simulink model "subsystem_118_bus"  (R2025b)
settings: Solver=ode45  StartTime=0.0  StopTime=Tstop  FixedStep=Ts  RelTol=1e-12  AbsTol=1e-12
values from neighbouring files (symbols this model uses):
  Imax = 15    [config_file.m]
  nominalInter =     [nominalInter.mat]
  nominalU =     [nominalU.mat]
  nominalY =     [nominalY.mat]
  sub = struct    [main_sub_118_bus.m]
  sys_j = sys_j(1:end-1)    [IBR_modelGenerator.m]
  sys_j_AA = sys_j    [modularMOR_main.m]
  sys_j_BT = sys_j    [modularMOR_main.m]
  Tstep_gfl = 0.1    [main_sub_118_bus.m]
  Tstep_gfm = 0.1    [main_sub_118_bus.m]
  w = 2*pi*50    (= 314.159265359)    [config_file.m]    (also in mirrorMimoWeightedFrequencyData.m = w(:); modularMOR_main.m = w(:).'; plotTest.m = w(:).')
undefined symbols (not defined in the file or in its folder): con_sub, linSys1, linSys2, linSys3
libraries: simulink x10
(part 3 of 6)

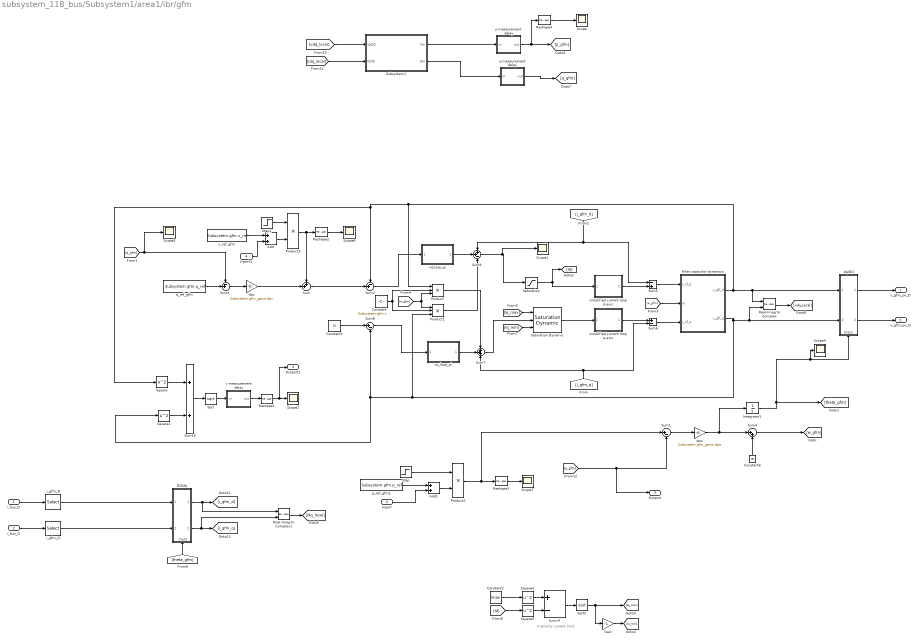
== system subsystem_118_bus/Subsystem1/area1/ibr/gfm ==
  note: P-priority current limit
  i_bus_D : Inport
  i_bus_Q : Inport  Port=2
  Inport : Inport  Port=3
  Inport1 : Inport  Port=4
  Add : Sum
  Add1 : Sum
  Constant : Constant  Value=Subsystem.gfm.c
  Constant1 : Constant  Value=0
  Constant2 : Constant  Value=Imax
  Constant6 : Constant  Value=w
  DQ/dq : Subsystem
      settings: PortSchema="{\"entries\":[{\"content\":{\"sides\":[{\"content\":{\"connectorIds\":[\"In1\",\"In2\"]},\"type\":\"ConnectorPlacement.EquallySpacedRectSide\",\"uuid\":\"6aba5a73-e9d3-440a-9da8-5b4060b79a22\"},{\"content\":{\"connectorIds\":[\"Out1\",\"Out2\"],\"side\":\"RIGHT\"},\"type\":\"ConnectorPlacement.EquallySpacedRectSide\",\"uuid\":\"fb100e33-0f2b-446b-b234-6a01cff1cf94\"},{\"content\":{\"connectorIds\":[],\"side\":\"TOP\"},\"type\":\"ConnectorPlacement.EquallySpacedRectSide\",\"uuid\":\"cb346bab-8363-4920-b8bd-1af08716b150\"},{\"content\":{\"connectorIds\":[\"In3\"],\"side\":\"BOTTOM\"},\"type\":\"ConnectorPlacement.EquallySpacedRectSide\",\"uuid\":\"daf67601-a33f-44c6-bbbf-d32eadf086e5\"},{\"content\":{\"connectorIds\":[],\"side\":\"HIDDEN\"},\"type\":\"ConnectorPlacement.EquallySpacedRectSide\",\"uuid\":\"157b31a2-d1ec-4854-8b21-1495795af5ef\"}]},\"type\":\"ConnectorPlacement.EquallySpacedConnector\",\"uuid\":\"bdcd0df2-60ef-4202-9e13-560935cf5e64\"}],\"packageUris\":[\"http://schema.mathworks.com/mf0/Connector/R2020b\"],\"version\":\"1.0\"}"
      mask Display: image('$imagefile'); % Use "Edit Image" on toolstrip to change.
  Gain : Gain  Gain=-1
  Integrator1 : Integrator  InitialCondition=Subsystem.gfm.theta  ContinuousStateAttributes='gfm_osc'
  Product : Product  Inputs=3
  Product1 : Product  Inputs=3
  Product2 : Product
  Product3 : Product
  Real-Imag to Complex : RealImagToComplex
  Real-Imag to Complex1 : RealImagToComplex
  Reshape{1..4} (4 alike) : Reshape
  Saturation : Saturate  UpperLimit=Imax  LowerLimit=-Imax
  Saturation Dynamic : simulink/Discontinuities/Saturation Dynamic  OutMin=[]  OutMax=[]  OutDataTypeStr=Inherit: Same as second input  OutDataType=fixdt(1, 16)  OutScaling=2^-10  DoSatur=off
  Scope{,1..2,4..5,7..8} (7 alike) : Scope
      Scope settings: ActiveDisplayYMinimum=-1  ActiveDisplayYMaximum=1  DataLoggingVariableName=pm_gfm  DataLoggingSaveFormat=Structure
      Scope1 settings: ActiveDisplayYMinimum=0.57567  ActiveDisplayYMaximum=1.70344
      Scope2 settings: ActiveDisplayYMinimum=1.02215  ActiveDisplayYMaximum=1.04295  DataLoggingVariableName=vm_gfm  DataLoggingSaveFormat=Structure
      Scope4 settings: ActiveDisplayYMinimum=-1  ActiveDisplayYMaximum=1  DataLoggingVariableName=thetagfmwnd  DataLoggingSaveFormat=Structure
      Scope5 settings: ActiveDisplayYMinimum=0.85975274896238685  ActiveDisplayYMaximum=1.0032219511840634  DataLoggingVariableName=qgfmwnd  DataLoggingSaveFormat=Structure
      Scope7 settings: ActiveDisplayYMinimum=-1  ActiveDisplayYMaximum=1  DataLoggingVariableName=pr_gfm  DataLoggingSaveFormat=Structure
      Scope8 settings: ActiveDisplayYMinimum=0.040000000000000036  ActiveDisplayYMaximum=2.04  DataLoggingVariableName=vr_gfm  DataLoggingSaveFormat=Structure
  Sqrt : Sqrt
  Sqrt2 : Sqrt
  Square{,1,4..5} (4 alike) : Math  Operator=square
  Step : Step  Time=Tstep_gfm  Before=Subsystem.P_before_gfm  After=Subsystem.P_after_gfm
  Step1 : Step  Time=Tstep_gfm  Before=Subsystem.V_before_gfm  After=Subsystem.V_after_gfm
  Subsystem1 : Subsystem
      mask Display: image('$imagefile'); % Use "Edit Image" on toolstrip to change.
  Sum : Sum  Inputs=++|
  Sum1 : Sum  Inputs=|+-
  Sum10 : Sum
  Sum14 : Sum  Inputs=+-
  Sum2 : Sum  Inputs=-+|
  Sum3 : Sum  Inputs=-+|
  Sum4 : Sum  Inputs=|++
  Sum5 : Sum  Inputs=-+
  Sum6 : Sum  Inputs=+-
  Sum7 : Sum  Inputs=+++
  Sum8 : Sum  Inputs=|+-
  Sum9 : Sum  Inputs=++-
  dpw : Gain  Gain=Subsystem.gfm_gains.dpw
  dq/DQ : Subsystem
      settings: PortSchema="{\"entries\":[{\"content\":{\"sides\":[{\"content\":{\"connectorIds\":[\"In1\",\"In2\"]},\"type\":\"ConnectorPlacement.EquallySpacedRectSide\",\"uuid\":\"6aba5a73-e9d3-440a-9da8-5b4060b79a22\"},{\"content\":{\"connectorIds\":[\"Out1\",\"Out2\"],\"side\":\"RIGHT\"},\"type\":\"ConnectorPlacement.EquallySpacedRectSide\",\"uuid\":\"fb100e33-0f2b-446b-b234-6a01cff1cf94\"},{\"content\":{\"connectorIds\":[],\"side\":\"TOP\"},\"type\":\"ConnectorPlacement.EquallySpacedRectSide\",\"uuid\":\"cb346bab-8363-4920-b8bd-1af08716b150\"},{\"content\":{\"connectorIds\":[\"In3\"],\"side\":\"BOTTOM\"},\"type\":\"ConnectorPlacement.EquallySpacedRectSide\",\"uuid\":\"daf67601-a33f-44c6-bbbf-d32eadf086e5\"},{\"content\":{\"connectorIds\":[],\"side\":\"HIDDEN\"},\"type\":\"ConnectorPlacement.EquallySpacedRectSide\",\"uuid\":\"157b31a2-d1ec-4854-8b21-1495795af5ef\"}]},\"type\":\"ConnectorPlacement.EquallySpacedConnector\",\"uuid\":\"bdcd0df2-60ef-4202-9e13-560935cf5e64\"}],\"packageUris\":[\"http://schema.mathworks.com/mf0/Connector/R2020b\"],\"version\":\"1.0\"}"
      mask Display: image('$imagefile'); % Use "Edit Image" on toolstrip to change.
  dqv : Gain  Gain=Subsystem.gfm_gains.dqv
  filter capacitor dynamics : Subsystem
      mask Display: image('$imagefile'); % Use "Edit Image" on toolstrip to change.
  i_gfm_D : Selector  InputPortWidth=size(Subsystem.sys_data,1)  IndexOptions=Index vector (dialog)  Indices=Subsystem.busnum.gfm  OutputSizes=1
  i_gfm_Q : Selector  InputPortWidth=size(Subsystem.sys_data,1)  IndexOptions=Index vector (dialog)  Indices=Subsystem.busnum.gfm  OutputSizes=1
  p measurement delay : Subsystem
      mask Display: image('$imagefile'); % Use "Edit Image" on toolstrip to change.
  p_ref_gfm1 : Constant  Value=Subsystem.gfm.p_ref
  q measurement delay : Subsystem
      mask Display: image('$imagefile'); % Use "Edit Image" on toolstrip to change.
  q_ref_gfm : Constant  Value=Subsystem.gfm.q_ref
  simplified current loop d-axis : Subsystem
      mask Display: image('$imagefile'); % Use "Edit Image" on toolstrip to change.
  simplified current loop q-axis : Subsystem
      mask Display: image('$imagefile'); % Use "Edit Image" on toolstrip to change.
  v measurement delay : Subsystem
      mask Display: image('$imagefile'); % Use "Edit Image" on toolstrip to change.
  v_ref_gfm : Constant  Value=Subsystem.gfm.v_ref
  vd_loop_pi : Subsystem
      mask Display: image('$imagefile'); % Use "Edit Image" on toolstrip to change.
  vq_loop_pi : Subsystem
      mask Display: image('$imagefile'); % Use "Edit Image" on toolstrip to change.
  v_gfm_pv_D : Outport
  v_gfm_pv_Q : Outport  Port=2
  Outport : Outport  Port=3
  Outport1 : Outport  Port=4
  wires:
  Sum2/1 -> vd_loop_pi/1("  ")
  dq/DQ/1(D-quantity) -> v_gfm_pv_D/1
  dq/DQ/2(Q-quantity) -> v_gfm_pv_Q/1
  dpw/1 -> Sum4/1, Integrator1/1
  [p_gfm] -> Outport/1, Sum1/2
  Constant6/1 -> Sum4/2
  Sum1/1 -> dpw/1
  Integrator1/1 -> [theta_gfm], Scope4/1, dq/DQ/3(theta)
  Sum/1 -> Sum2/2
  dqv/1 -> Sum/2
  Sum3/1 -> dqv/1
  q_ref_gfm/1 -> Sum3/2
  [q_gfm] -> Sum3/1, Scope5/1
  Sum6/1 -> filter capacitor dynamics/3(i_cf_q)
  simplified current loop q-axis/1("  ") -> Sum6/1
  Sum5/1 -> filter capacitor dynamics/1(i_cf_d)
  [theta_gfm] -> DQ/dq/3(theta)
  vq_loop_pi/1(" ") -> Sum7/2
  Sum8/1 -> vq_loop_pi/1("  ")
  vd_loop_pi/1(" ") -> Sum9/2
  [i_gfm_q] -> Sum6/2, Sum7/3
  [i_gfm_d] -> Sum5/1, Sum9/1
  Product/1 -> Sum7/1
  Product1/1 -> Sum9/3
  Sum4/1 -> [w_gfm]
  [w_gfm] -> filter capacitor dynamics/2(w)
  [w_gfm] -> Product/3, Product1/1
  Constant/1 -> Product1/2, Product/2
  Constant1/1 -> Sum8/1
  simplified current loop d-axis/1("  ") -> Sum5/2
  Square/1 -> Sum10/1
  Square1/1 -> Sum10/2
  Sum10/1 -> Sqrt/1
  Sqrt/1 -> v measurement delay/1(in)
  v measurement delay/1(out) -> Reshape1/1
  Product2/1 -> Sum1/1, Reshape3/1
  Step/1 -> Product2/1
  Step1/1 -> Product3/1
  Product3/1 -> Reshape2/1, Sum/1
  Sum7/1 -> Saturation Dynamic/2
  [Iq_max] -> Saturation Dynamic/1
  [Iq_min] -> Saturation Dynamic/3
  Saturation/1 -> simplified current loop d-axis/1(" "), [Id]
  Saturation Dynamic/1 -> simplified current loop q-axis/1(" ")
  Sum9/1 -> Scope1/1, Saturation/1
  Square5/1 -> Sum14/2
  Sum14/1 -> Sqrt2/1
  Sqrt2/1 -> [Iq_max], Gain/1
  Constant2/1 -> Square4/1
  Gain/1 -> [Iq_min]
  Square4/1 -> Sum14/1
  [Id] -> Square5/1
  i_bus_Q/1 -> i_gfm_Q/1
  i_bus_D/1 -> i_gfm_D/1
  i_gfm_D/1 -> DQ/dq/1(D_quantity)
  i_gfm_Q/1 -> DQ/dq/2(Q_quantity)
  Subsystem1/1(Pm) -> p measurement delay/1(in)
  Reshape4/1 -> Scope/1
  p measurement delay/1(out) -> [p_gfm], Reshape4/1
  [vdq_local] -> Subsystem1/1(vbDQ)
  [idq_local] -> Subsystem1/2(IbDQ)
  Real-Imag to Complex1/1 -> [idq_local]
  DQ/dq/2(q_quantity) -> Real-Imag to Complex1/2, [i_gfm_q]
  DQ/dq/1(d_quantity) -> Real-Imag to Complex1/1, [i_gfm_d]
  filter capacitor dynamics/2(v_gfl_q) -> Real-Imag to Complex/2, dq/DQ/2(q-quantity), Product1/3, Square1/1, Sum8/2
  Real-Imag to Complex/1 -> [vdq_local]
  filter capacitor dynamics/1(v_gfl_d) -> Real-Imag to Complex/1, dq/DQ/1(d-quantity), Product/1, Sum2/1, Square/1
  Subsystem1/2(Qm) -> q measurement delay/1(in)
  q measurement delay/1(out) -> [q_gfm]
  Reshape2/1 -> Scope8/1
  Reshape3/1 -> Scope7/1
  Reshape1/1 -> Outport1/1, Scope2/1
  Add/1 -> Product3/2
  v_ref_gfm/1 -> Add/1
  Add1/1 -> Product2/2
  p_ref_gfm1/1 -> Add1/1
  Inport/1 -> Add1/2
  Inport1/1 -> Add/2

== system subsystem_118_bus/Subsystem1/area1/non_ibr/floating buses ==
  In1 : Inport
  In2 : Inport  Port=2
  i_float_D : Selector  InputPortWidth=size(Subsystem.sys_data,1)  IndexOptions=Index vector (dialog)  Indices=Subsystem.busnum.float  OutputSizes=1
  i_float_Q : Selector  InputPortWidth=size(Subsystem.sys_data,1)  IndexOptions=Index vector (dialog)  Indices=Subsystem.busnum.float  OutputSizes=1
  line charging dynamics : Subsystem
      mask Display: image('$imagefile'); % Use "Edit Image" on toolstrip to change.
  v_float_D : Outport
  v_float_Q : Outport  Port=2
  wires:
  i_float_D/1 -> line charging dynamics/1(i_float_D)
  In2/1 -> i_float_Q/1
  i_float_Q/1 -> line charging dynamics/2(i_float_Q)
  In1/1 -> i_float_D/1
  line charging dynamics/2(v_float_Q) -> v_float_Q/1
  line charging dynamics/1(v_float_D) -> v_float_D/1

== system subsystem_118_bus/Subsystem1/area1/non_ibr/infinite bus ==
  v_inf_D : Constant  Value=Subsystem.infbus.v_D
  v_inf_Q : Constant  Value=Subsystem.infbus.v_Q
  Out1 : Outport
  Out2 : Outport  Port=2
  wires:
  v_inf_Q/1 -> Out2/1
  v_inf_D/1 -> Out1/1

== system subsystem_118_bus/Subsystem1/area1/non_ibr/load buses ==
  In1 : Inport
  In2 : Inport  Port=2
  Constant : Constant  Value=Subsystem.load1.v_D
  Constant1 : Constant  Value=Subsystem.load1.v_Q
  Constant2 : Constant  Value=Subsystem.load1.ptype
  Constant3 : Constant  Value=Subsystem.load1.qtype
  Divide : Product  Inputs=*/
  Product : Product
  Product1 : Product
  Sqrt : Sqrt
  Sqrt1 : Sqrt
  Square1 : Math  Operator=pow
  Square{2..5} (4 alike) : Math  Operator=square
  Square6 : Math  Operator=pow
  Subsystem : Subsystem
  Sum : Sum  Inputs=|-+
  Sum1 : Sum  Inputs=|-+
  Sum2 : Sum
  Sum4 : Sum
  i_load_D : Selector  InputPortWidth=size(Subsystem.sys_data,1)  IndexOptions=Index vector (dialog)  Indices=Subsystem.busnum.load  OutputSizes=1
  i_load_Q : Selector  InputPortWidth=size(Subsystem.sys_data,1)  IndexOptions=Index vector (dialog)  Indices=Subsystem.busnum.load  OutputSizes=1
  line charging dynamics : Subsystem
      mask Display: image('$imagefile'); % Use "Edit Image" on toolstrip to change.
  load bus p : Constant  Value=Subsystem.load1.p
  load bus q : Constant  Value=Subsystem.load1.q
  Out1 : Outport
  Out2 : Outport  Port=2
  wires:
  In1/1 -> i_load_D/1
  In2/1 -> i_load_Q/1
  Sum1/1 -> line charging dynamics/2(i_load_c_Q)
  i_load_Q/1 -> Sum1/1
  i_load_D/1 -> Sum/1
  [v_load_D] -> Subsystem/3(vD)
  [v_load_Q] -> Subsystem/4(vQ)
  Subsystem/2(i_inj_load_q) -> Sum1/2
  Subsystem/1(i_inj_load_d) -> Sum/2
  Sum/1 -> line charging dynamics/1(i_load_c_D)
  load bus p/1 -> Product/1
  Square6/1 -> Product/2
  Product/1 -> Subsystem/1(p)
  Product1/1 -> Subsystem/2(q)
  load bus q/1 -> Product1/2
  line charging dynamics/1(v_load_D) -> Out1/1, [v_load_D]
  line charging dynamics/2(v_load_Q) -> Out2/1, [v_load_Q]
  Square1/1 -> Product1/1
  Sum2/1 -> Sqrt1/1
  Square4/1 -> Sum2/1
  Constant1/1 -> Square3/1
  [v_load_D] -> Square4/1
  Square5/1 -> Sum2/2
  Constant2/1 -> Square6/2
  Divide/1 -> Square6/1, Square1/1
  Constant/1 -> Square2/1
  Sqrt/1 -> Divide/2
  Square3/1 -> Sum4/2
  Sqrt1/1 -> Divide/1
  Sum4/1 -> Sqrt/1
  Square2/1 -> Sum4/1
  [v_load_Q] -> Square5/1
  Constant3/1 -> Square1/2

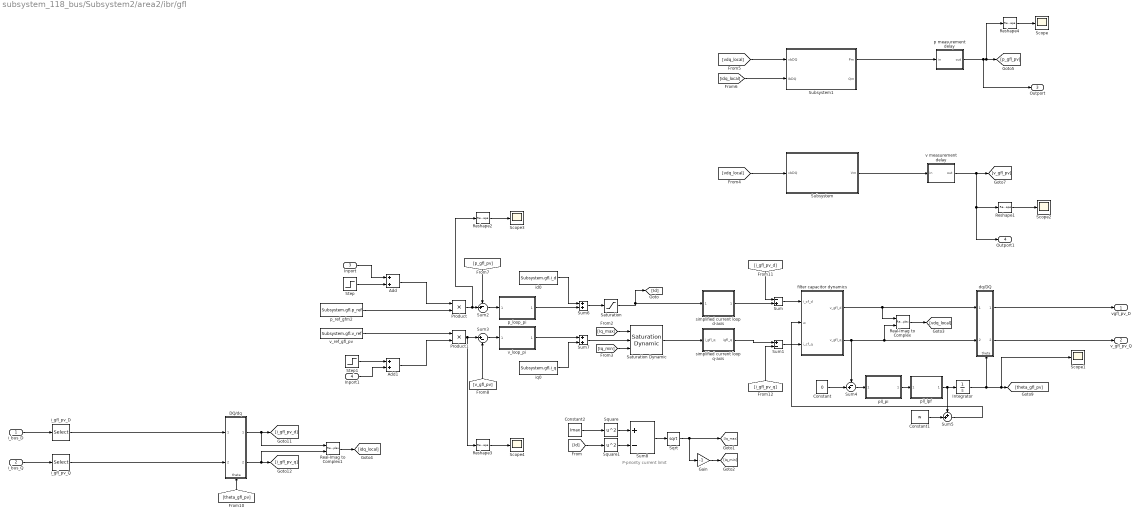
== system subsystem_118_bus/Subsystem2/area2/ibr/gfl ==
  note: P-priority current limit
  i_bus_D : Inport
  i_bus_Q : Inport  Port=2
  Inport : Inport  Port=3
  Inport1 : Inport  Port=4
  Add : Sum
  Add1 : Sum
  Constant : Constant  Value=0
  Constant1 : Constant  Value=w
  Constant2 : Constant  Value=Imax
  DQ/dq : Subsystem
      settings: PortSchema="{\"entries\":[{\"content\":{\"sides\":[{\"content\":{\"connectorIds\":[\"In1\",\"In2\"]},\"type\":\"ConnectorPlacement.EquallySpacedRectSide\",\"uuid\":\"6aba5a73-e9d3-440a-9da8-5b4060b79a22\"},{\"content\":{\"connectorIds\":[\"Out1\",\"Out2\"],\"side\":\"RIGHT\"},\"type\":\"ConnectorPlacement.EquallySpacedRectSide\",\"uuid\":\"fb100e33-0f2b-446b-b234-6a01cff1cf94\"},{\"content\":{\"connectorIds\":[],\"side\":\"TOP\"},\"type\":\"ConnectorPlacement.EquallySpacedRectSide\",\"uuid\":\"cb346bab-8363-4920-b8bd-1af08716b150\"},{\"content\":{\"connectorIds\":[\"In3\"],\"side\":\"BOTTOM\"},\"type\":\"ConnectorPlacement.EquallySpacedRectSide\",\"uuid\":\"daf67601-a33f-44c6-bbbf-d32eadf086e5\"},{\"content\":{\"connectorIds\":[],\"side\":\"HIDDEN\"},\"type\":\"ConnectorPlacement.EquallySpacedRectSide\",\"uuid\":\"157b31a2-d1ec-4854-8b21-1495795af5ef\"}]},\"type\":\"ConnectorPlacement.EquallySpacedConnector\",\"uuid\":\"bdcd0df2-60ef-4202-9e13-560935cf5e64\"}],\"packageUris\":[\"http://schema.mathworks.com/mf0/Connector/R2020b\"],\"version\":\"1.0\"}"
      mask Display: image('$imagefile'); % Use "Edit Image" on toolstrip to change.
  Gain : Gain  Gain=-1
  Integrator : Integrator  InitialCondition=Subsystem.gfl.theta  ContinuousStateAttributes='gfl_osc'
  Product : Product
  Product1 : Product
  Real-Imag to Complex : RealImagToComplex
  Real-Imag to Complex1 : RealImagToComplex
  Reshape{1..4} (4 alike) : Reshape
  Saturation : Saturate  UpperLimit=Imax  LowerLimit=-Imax
  Saturation Dynamic : simulink/Discontinuities/Saturation Dynamic  OutMin=[]  OutMax=[]  OutDataTypeStr=Inherit: Same as second input  OutDataType=fixdt(1, 16)  OutScaling=2^-10  DoSatur=off
  Scope{,1..4} (5 alike) : Scope
      Scope settings: ActiveDisplayYMinimum=-1  ActiveDisplayYMaximum=1  DataLoggingVariableName=pm_gfl  DataLoggingSaveFormat=Structure
      Scope1 settings: DataLoggingVariableName=thetagflwnd  DataLoggingSaveFormat=Structure
      Scope2 settings: ActiveDisplayYMinimum=-1  ActiveDisplayYMaximum=1  DataLoggingVariableName=vm_gfl  DataLoggingSaveFormat=Structure
      Scope3 settings: ActiveDisplayYMinimum=0.75  ActiveDisplayYMaximum=0.95  DataLoggingVariableName=pr_gfl  DataLoggingSaveFormat=Structure
      Scope4 settings: ActiveDisplayYMinimum=1.02188  ActiveDisplayYMaximum=1.05312  DataLoggingVariableName=vr_gfl  DataLoggingSaveFormat=Structure
  Sqrt : Sqrt
  Square : Math  Operator=square
  Square1 : Math  Operator=square
  Step : Step  Time=Tstep_gfl  Before=Subsystem.P_before_gfl  After=Subsystem.P_after_gfl  SampleTime=0
  Step1 : Step  Time=Tstep_gfl  Before=Subsystem.V_before_gfl  After=Subsystem.V_after_gfl  SampleTime=0
  Subsystem : Subsystem
      mask Display: image('$imagefile'); % Use "Edit Image" on toolstrip to change.
  Subsystem1 : Subsystem
      mask Display: image('$imagefile'); % Use "Edit Image" on toolstrip to change.
  Sum : Sum  Inputs=-+
  Sum1 : Sum  Inputs=+-
  Sum2 : Sum  Inputs=-+|
  Sum3 : Sum  Inputs=|+-
  Sum4 : Sum  Inputs=-+|
  Sum5 : Sum  Inputs=++|
  Sum6 : Sum
  Sum7 : Sum
  Sum8 : Sum  Inputs=+-
  dq/DQ : Subsystem
      settings: PortSchema="{\"entries\":[{\"content\":{\"sides\":[{\"content\":{\"connectorIds\":[\"In1\",\"In2\"]},\"type\":\"ConnectorPlacement.EquallySpacedRectSide\",\"uuid\":\"6aba5a73-e9d3-440a-9da8-5b4060b79a22\"},{\"content\":{\"connectorIds\":[\"Out1\",\"Out2\"],\"side\":\"RIGHT\"},\"type\":\"ConnectorPlacement.EquallySpacedRectSide\",\"uuid\":\"fb100e33-0f2b-446b-b234-6a01cff1cf94\"},{\"content\":{\"connectorIds\":[],\"side\":\"TOP\"},\"type\":\"ConnectorPlacement.EquallySpacedRectSide\",\"uuid\":\"cb346bab-8363-4920-b8bd-1af08716b150\"},{\"content\":{\"connectorIds\":[\"In3\"],\"side\":\"BOTTOM\"},\"type\":\"ConnectorPlacement.EquallySpacedRectSide\",\"uuid\":\"daf67601-a33f-44c6-bbbf-d32eadf086e5\"},{\"content\":{\"connectorIds\":[],\"side\":\"HIDDEN\"},\"type\":\"ConnectorPlacement.EquallySpacedRectSide\",\"uuid\":\"157b31a2-d1ec-4854-8b21-1495795af5ef\"}]},\"type\":\"ConnectorPlacement.EquallySpacedConnector\",\"uuid\":\"bdcd0df2-60ef-4202-9e13-560935cf5e64\"}],\"packageUris\":[\"http://schema.mathworks.com/mf0/Connector/R2020b\"],\"version\":\"1.0\"}"
      mask Display: image('$imagefile'); % Use "Edit Image" on toolstrip to change.
  filter capacitor dynamics : Subsystem
      mask Display: image('$imagefile'); % Use "Edit Image" on toolstrip to change.
  i_gfl_pv_D : Selector  InputPortWidth=size(Subsystem.sys_data,1)  IndexOptions=Index vector (dialog)  Indices=Subsystem.busnum.gfl  OutputSizes=1
  i_gfl_pv_Q : Selector  InputPortWidth=size(Subsystem.sys_data,1)  IndexOptions=Index vector (dialog)  Indices=Subsystem.busnum.gfl  OutputSizes=1
  id0 : Constant  Value=Subsystem.gfl.i_d
  iq0 : Constant  Value=Subsystem.gfl.i_q
  p measurement delay : Subsystem
      mask Display: image('$imagefile'); % Use "Edit Image" on toolstrip to change.
  p_loop_pi : Subsystem
      mask Display: image('$imagefile'); % Use "Edit Image" on toolstrip to change.
  p_ref_gfm2 : Constant  Value=Subsystem.gfl.p_ref
  pll_lpf : Subsystem
      mask Display: image('$imagefile'); % Use "Edit Image" on toolstrip to change.
  pll_pi : Subsystem
      mask Display: image('$imagefile'); % Use "Edit Image" on toolstrip to change.
  simplified current loop d-axis : Subsystem
      mask Display: image('$imagefile'); % Use "Edit Image" on toolstrip to change.
  simplified current loop q-axis : Subsystem
      mask Display: image('$imagefile'); % Use "Edit Image" on toolstrip to change.
  v measurement delay : Subsystem
      mask Display: image('$imagefile'); % Use "Edit Image" on toolstrip to change.
  v_loop_pi : Subsystem
      mask Display: image('$imagefile'); % Use "Edit Image" on toolstrip to change.
  v_ref_gfl_pv : Constant  Value=Subsystem.gfl.v_ref
  vgfl_pv_D : Outport
  v_gfl_pv_Q : Outport  Port=2
  Outport : Outport  Port=3
  Outport1 : Outport  Port=4
  wires:
  pll_lpf/1(LPF_output) -> Sum5/1, Integrator/1
  Constant/1 -> Sum4/2
  filter capacitor dynamics/1(v_gfl_d) -> dq/DQ/1(d-quantity), Real-Imag to Complex/1
  v measurement delay/1(out) -> Reshape1/1, Outport1/1, [v_gfl_pv]
  filter capacitor dynamics/2(v_gfl_q) -> Real-Imag to Complex/2, dq/DQ/2(q-quantity), Sum4/1
  [p_gfl_pv] -> Sum2/1
  Sum1/1 -> filter capacitor dynamics/3(i_cf_q)
  Sum4/1 -> pll_pi/1("  ")
  Sum5/1 -> filter capacitor dynamics/2(w)
  dq/DQ/1(D-quantity) -> vgfl_pv_D/1
  Sum2/1 -> p_loop_pi/1("  ")
  p measurement delay/1(out) -> Outport/1, Reshape4/1, [p_gfl_pv]
  Constant1/1 -> Sum5/2
  Sum3/1 -> v_loop_pi/1("  ")
  [i_gfl_pv_d] -> Sum/1
  Sum/1 -> filter capacitor dynamics/1(i_cf_d)
  [i_gfl_pv_q] -> Sum1/2
  [theta_gfl_pv] -> DQ/dq/3(theta)
  pll_pi/1(" ") -> pll_lpf/1(LPF_input)
  [v_gfl_pv] -> Sum3/2
  i_bus_Q/1 -> i_gfl_pv_Q/1
  i_bus_D/1 -> i_gfl_pv_D/1
  p_loop_pi/1(" ") -> Sum6/2
  v_loop_pi/1(" ") -> Sum7/1
  iq0/1 -> Sum7/2
  id0/1 -> Sum6/1
  Sum6/1 -> Saturation/1
  Integrator/1 -> Scope1/1, [theta_gfl_pv], dq/DQ/3(theta)
  Reshape4/1 -> Scope/1
  Reshape1/1 -> Scope2/1
  [Id] -> Square1/1
  Gain/1 -> [Iq_min]
  Constant2/1 -> Square/1
  Square/1 -> Sum8/1
  Sqrt/1 -> [Iq_max], Gain/1
  Square1/1 -> Sum8/2
  Sum8/1 -> Sqrt/1
  Saturation/1 -> simplified current loop d-axis/1(" "), [Id]
  Sum7/1 -> Saturation Dynamic/2
  [Iq_max] -> Saturation Dynamic/1
  [Iq_min] -> Saturation Dynamic/3
  simplified current loop d-axis/1("  ") -> Sum/2
  Saturation Dynamic/1 -> simplified current loop q-axis/1(i_gfl_q)
  simplified current loop q-axis/1(igfl_q) -> Sum1/1
  [vdq_local] -> Subsystem/1(vbDQ)
  [vdq_local] -> Subsystem1/1(vbDQ)
  [idq_local] -> Subsystem1/2(IbDQ)
  Real-Imag to Complex/1 -> [vdq_local]
  DQ/dq/1(d_quantity) -> Real-Imag to Complex1/1, [i_gfl_pv_d]
  DQ/dq/2(q_quantity) -> Real-Imag to Complex1/2, [i_gfl_pv_q]
  Real-Imag to Complex1/1 -> [idq_local]
  dq/DQ/2(Q-quantity) -> v_gfl_pv_Q/1
  Subsystem/1(Vm) -> v measurement delay/1(in)
  Subsystem1/1(Pm) -> p measurement delay/1(in)
  p_ref_gfm2/1 -> Product/2
  v_ref_gfl_pv/1 -> Product1/1
  Reshape2/1 -> Scope3/1
  Product/1 -> Reshape2/1, Sum2/2
  Reshape3/1 -> Scope4/1
  Product1/1 -> Sum3/1, Reshape3/1
  Step/1 -> Add/2
  Add/1 -> Product/1
  Step1/1 -> Add1/1
  Add1/1 -> Product1/2
  Inport/1 -> Add/1
  Inport1/1 -> Add1/2
  i_gfl_pv_D/1 -> DQ/dq/1(D_quantity)
  i_gfl_pv_Q/1 -> DQ/dq/2(Q_quantity)

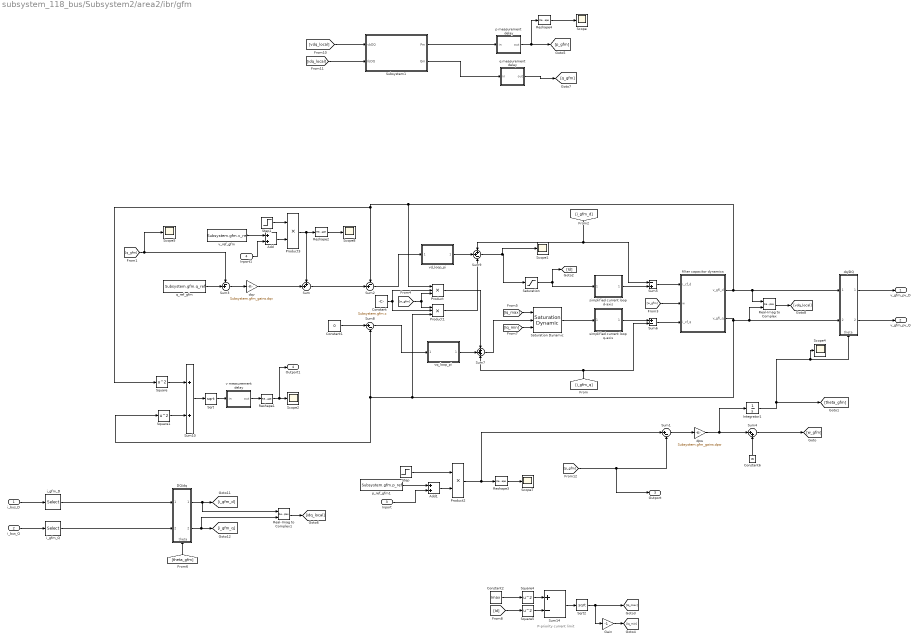
== system subsystem_118_bus/Subsystem2/area2/ibr/gfm ==
  note: P-priority current limit
  i_bus_D : Inport
  i_bus_Q : Inport  Port=2
  Inport : Inport  Port=3
  Inport1 : Inport  Port=4
  Add : Sum
  Add1 : Sum
  Constant : Constant  Value=Subsystem.gfm.c
  Constant1 : Constant  Value=0
  Constant2 : Constant  Value=Imax
  Constant6 : Constant  Value=w
  DQ/dq : Subsystem
      settings: PortSchema="{\"entries\":[{\"content\":{\"sides\":[{\"content\":{\"connectorIds\":[\"In1\",\"In2\"]},\"type\":\"ConnectorPlacement.EquallySpacedRectSide\",\"uuid\":\"6aba5a73-e9d3-440a-9da8-5b4060b79a22\"},{\"content\":{\"connectorIds\":[\"Out1\",\"Out2\"],\"side\":\"RIGHT\"},\"type\":\"ConnectorPlacement.EquallySpacedRectSide\",\"uuid\":\"fb100e33-0f2b-446b-b234-6a01cff1cf94\"},{\"content\":{\"connectorIds\":[],\"side\":\"TOP\"},\"type\":\"ConnectorPlacement.EquallySpacedRectSide\",\"uuid\":\"cb346bab-8363-4920-b8bd-1af08716b150\"},{\"content\":{\"connectorIds\":[\"In3\"],\"side\":\"BOTTOM\"},\"type\":\"ConnectorPlacement.EquallySpacedRectSide\",\"uuid\":\"daf67601-a33f-44c6-bbbf-d32eadf086e5\"},{\"content\":{\"connectorIds\":[],\"side\":\"HIDDEN\"},\"type\":\"ConnectorPlacement.EquallySpacedRectSide\",\"uuid\":\"157b31a2-d1ec-4854-8b21-1495795af5ef\"}]},\"type\":\"ConnectorPlacement.EquallySpacedConnector\",\"uuid\":\"bdcd0df2-60ef-4202-9e13-560935cf5e64\"}],\"packageUris\":[\"http://schema.mathworks.com/mf0/Connector/R2020b\"],\"version\":\"1.0\"}"
      mask Display: image('$imagefile'); % Use "Edit Image" on toolstrip to change.
  Gain : Gain  Gain=-1
  Integrator1 : Integrator  InitialCondition=Subsystem.gfm.theta  ContinuousStateAttributes='gfm_osc'
  Product : Product  Inputs=3
  Product1 : Product  Inputs=3
  Product2 : Product
  Product3 : Product
  Real-Imag to Complex : RealImagToComplex
  Real-Imag to Complex1 : RealImagToComplex
  Reshape{1..4} (4 alike) : Reshape
  Saturation : Saturate  UpperLimit=Imax  LowerLimit=-Imax
  Saturation Dynamic : simulink/Discontinuities/Saturation Dynamic  OutMin=[]  OutMax=[]  OutDataTypeStr=Inherit: Same as second input  OutDataType=fixdt(1, 16)  OutScaling=2^-10  DoSatur=off
  Scope{,1..2,4..5,7..8} (7 alike) : Scope
      Scope settings: ActiveDisplayYMinimum=-1  ActiveDisplayYMaximum=1  DataLoggingVariableName=pm_gfm  DataLoggingSaveFormat=Structure
      Scope1 settings: ActiveDisplayYMinimum=0.57567  ActiveDisplayYMaximum=1.70344
      Scope2 settings: ActiveDisplayYMinimum=1.02215  ActiveDisplayYMaximum=1.04295  DataLoggingVariableName=vm_gfm  DataLoggingSaveFormat=Structure
      Scope4 settings: ActiveDisplayYMinimum=-1  ActiveDisplayYMaximum=1  DataLoggingVariableName=thetagfmwnd  DataLoggingSaveFormat=Structure
      Scope5 settings: ActiveDisplayYMinimum=0.85975274896238685  ActiveDisplayYMaximum=1.0032219511840634  DataLoggingVariableName=qgfmwnd  DataLoggingSaveFormat=Structure
      Scope7 settings: ActiveDisplayYMinimum=-1  ActiveDisplayYMaximum=1  DataLoggingVariableName=pr_gfm  DataLoggingSaveFormat=Structure
      Scope8 settings: ActiveDisplayYMinimum=0.040000000000000036  ActiveDisplayYMaximum=2.04  DataLoggingVariableName=vr_gfm  DataLoggingSaveFormat=Structure
  Sqrt : Sqrt
  Sqrt2 : Sqrt
  Square{,1,4..5} (4 alike) : Math  Operator=square
  Step : Step  Time=Tstep_gfm  Before=Subsystem.P_before_gfm  After=Subsystem.P_after_gfm
  Step1 : Step  Time=Tstep_gfm  Before=Subsystem.V_before_gfm  After=Subsystem.V_after_gfm
  Subsystem1 : Subsystem
      mask Display: image('$imagefile'); % Use "Edit Image" on toolstrip to change.
  Sum : Sum  Inputs=++|
  Sum1 : Sum  Inputs=|+-
  Sum10 : Sum
  Sum14 : Sum  Inputs=+-
  Sum2 : Sum  Inputs=-+|
  Sum3 : Sum  Inputs=-+|
  Sum4 : Sum  Inputs=|++
  Sum5 : Sum  Inputs=-+
  Sum6 : Sum  Inputs=+-
  Sum7 : Sum  Inputs=+++
  Sum8 : Sum  Inputs=|+-
  Sum9 : Sum  Inputs=++-
  dpw : Gain  Gain=Subsystem.gfm_gains.dpw
  dq/DQ : Subsystem
      settings: PortSchema="{\"entries\":[{\"content\":{\"sides\":[{\"content\":{\"connectorIds\":[\"In1\",\"In2\"]},\"type\":\"ConnectorPlacement.EquallySpacedRectSide\",\"uuid\":\"6aba5a73-e9d3-440a-9da8-5b4060b79a22\"},{\"content\":{\"connectorIds\":[\"Out1\",\"Out2\"],\"side\":\"RIGHT\"},\"type\":\"ConnectorPlacement.EquallySpacedRectSide\",\"uuid\":\"fb100e33-0f2b-446b-b234-6a01cff1cf94\"},{\"content\":{\"connectorIds\":[],\"side\":\"TOP\"},\"type\":\"ConnectorPlacement.EquallySpacedRectSide\",\"uuid\":\"cb346bab-8363-4920-b8bd-1af08716b150\"},{\"content\":{\"connectorIds\":[\"In3\"],\"side\":\"BOTTOM\"},\"type\":\"ConnectorPlacement.EquallySpacedRectSide\",\"uuid\":\"daf67601-a33f-44c6-bbbf-d32eadf086e5\"},{\"content\":{\"connectorIds\":[],\"side\":\"HIDDEN\"},\"type\":\"ConnectorPlacement.EquallySpacedRectSide\",\"uuid\":\"157b31a2-d1ec-4854-8b21-1495795af5ef\"}]},\"type\":\"ConnectorPlacement.EquallySpacedConnector\",\"uuid\":\"bdcd0df2-60ef-4202-9e13-560935cf5e64\"}],\"packageUris\":[\"http://schema.mathworks.com/mf0/Connector/R2020b\"],\"version\":\"1.0\"}"
      mask Display: image('$imagefile'); % Use "Edit Image" on toolstrip to change.
  dqv : Gain  Gain=Subsystem.gfm_gains.dqv
  filter capacitor dynamics : Subsystem
      mask Display: image('$imagefile'); % Use "Edit Image" on toolstrip to change.
  i_gfm_D : Selector  InputPortWidth=size(Subsystem.sys_data,1)  IndexOptions=Index vector (dialog)  Indices=Subsystem.busnum.gfm  OutputSizes=1
  i_gfm_Q : Selector  InputPortWidth=size(Subsystem.sys_data,1)  IndexOptions=Index vector (dialog)  Indices=Subsystem.busnum.gfm  OutputSizes=1
  p measurement delay : Subsystem
      mask Display: image('$imagefile'); % Use "Edit Image" on toolstrip to change.
  p_ref_gfm1 : Constant  Value=Subsystem.gfm.p_ref
  q measurement delay : Subsystem
      mask Display: image('$imagefile'); % Use "Edit Image" on toolstrip to change.
  q_ref_gfm : Constant  Value=Subsystem.gfm.q_ref
  simplified current loop d-axis : Subsystem
      mask Display: image('$imagefile'); % Use "Edit Image" on toolstrip to change.
  simplified current loop q-axis : Subsystem
      mask Display: image('$imagefile'); % Use "Edit Image" on toolstrip to change.
  v measurement delay : Subsystem
      mask Display: image('$imagefile'); % Use "Edit Image" on toolstrip to change.
  v_ref_gfm : Constant  Value=Subsystem.gfm.v_ref
  vd_loop_pi : Subsystem
      mask Display: image('$imagefile'); % Use "Edit Image" on toolstrip to change.
  vq_loop_pi : Subsystem
      mask Display: image('$imagefile'); % Use "Edit Image" on toolstrip to change.
  v_gfm_pv_D : Outport
  v_gfm_pv_Q : Outport  Port=2
  Outport : Outport  Port=3
  Outport1 : Outport  Port=4
  wires:
  Sum2/1 -> vd_loop_pi/1("  ")
  dq/DQ/1(D-quantity) -> v_gfm_pv_D/1
  dq/DQ/2(Q-quantity) -> v_gfm_pv_Q/1
  dpw/1 -> Sum4/1, Integrator1/1
  [p_gfm] -> Outport/1, Sum1/2
  Constant6/1 -> Sum4/2
  Sum1/1 -> dpw/1
  Integrator1/1 -> [theta_gfm], Scope4/1, dq/DQ/3(theta)
  Sum/1 -> Sum2/2
  dqv/1 -> Sum/2
  Sum3/1 -> dqv/1
  q_ref_gfm/1 -> Sum3/2
  [q_gfm] -> Sum3/1, Scope5/1
  Sum6/1 -> filter capacitor dynamics/3(i_cf_q)
  simplified current loop q-axis/1("  ") -> Sum6/1
  Sum5/1 -> filter capacitor dynamics/1(i_cf_d)
  [theta_gfm] -> DQ/dq/3(theta)
  vq_loop_pi/1(" ") -> Sum7/2
  Sum8/1 -> vq_loop_pi/1("  ")
  vd_loop_pi/1(" ") -> Sum9/2
  [i_gfm_q] -> Sum6/2, Sum7/3
  [i_gfm_d] -> Sum5/1, Sum9/1
  Product/1 -> Sum7/1
  Product1/1 -> Sum9/3
  Sum4/1 -> [w_gfm]
  [w_gfm] -> filter capacitor dynamics/2(w)
  [w_gfm] -> Product/3, Product1/1
  Constant/1 -> Product1/2, Product/2
  Constant1/1 -> Sum8/1
  simplified current loop d-axis/1("  ") -> Sum5/2
  Square/1 -> Sum10/1
  Square1/1 -> Sum10/2
  Sum10/1 -> Sqrt/1
  Sqrt/1 -> v measurement delay/1(in)
  v measurement delay/1(out) -> Reshape1/1
  Product2/1 -> Sum1/1, Reshape3/1
  Step/1 -> Product2/1
  Step1/1 -> Product3/1
  Product3/1 -> Reshape2/1, Sum/1
  Sum7/1 -> Saturation Dynamic/2
  [Iq_max] -> Saturation Dynamic/1
  [Iq_min] -> Saturation Dynamic/3
  Saturation/1 -> simplified current loop d-axis/1(" "), [Id]
  Saturation Dynamic/1 -> simplified current loop q-axis/1(" ")
  Sum9/1 -> Scope1/1, Saturation/1
  Square5/1 -> Sum14/2
  Sum14/1 -> Sqrt2/1
  Sqrt2/1 -> [Iq_max], Gain/1
  Constant2/1 -> Square4/1
  Gain/1 -> [Iq_min]
  Square4/1 -> Sum14/1
  [Id] -> Square5/1
  i_bus_Q/1 -> i_gfm_Q/1
  i_bus_D/1 -> i_gfm_D/1
  i_gfm_D/1 -> DQ/dq/1(D_quantity)
  i_gfm_Q/1 -> DQ/dq/2(Q_quantity)
  Subsystem1/1(Pm) -> p measurement delay/1(in)
  Reshape4/1 -> Scope/1
  p measurement delay/1(out) -> [p_gfm], Reshape4/1
  [vdq_local] -> Subsystem1/1(vbDQ)
  [idq_local] -> Subsystem1/2(IbDQ)
  Real-Imag to Complex1/1 -> [idq_local]
  DQ/dq/2(q_quantity) -> Real-Imag to Complex1/2, [i_gfm_q]
  DQ/dq/1(d_quantity) -> Real-Imag to Complex1/1, [i_gfm_d]
  filter capacitor dynamics/2(v_gfl_q) -> Real-Imag to Complex/2, dq/DQ/2(q-quantity), Product1/3, Square1/1, Sum8/2
  Real-Imag to Complex/1 -> [vdq_local]
  filter capacitor dynamics/1(v_gfl_d) -> Real-Imag to Complex/1, dq/DQ/1(d-quantity), Product/1, Sum2/1, Square/1
  Subsystem1/2(Qm) -> q measurement delay/1(in)
  q measurement delay/1(out) -> [q_gfm]
  Reshape2/1 -> Scope8/1
  Reshape3/1 -> Scope7/1
  Reshape1/1 -> Outport1/1, Scope2/1
  Add/1 -> Product3/2
  v_ref_gfm/1 -> Add/1
  Add1/1 -> Product2/2
  p_ref_gfm1/1 -> Add1/1
  Inport/1 -> Add1/2
  Inport1/1 -> Add/2

== system subsystem_118_bus/Subsystem2/area2/non_ibr/floating buses ==
  In1 : Inport
  In2 : Inport  Port=2
  i_float_D : Selector  InputPortWidth=size(Subsystem.sys_data,1)  IndexOptions=Index vector (dialog)  Indices=Subsystem.busnum.float  OutputSizes=1
  i_float_Q : Selector  InputPortWidth=size(Subsystem.sys_data,1)  IndexOptions=Index vector (dialog)  Indices=Subsystem.busnum.float  OutputSizes=1
  line charging dynamics : Subsystem
      mask Display: image('$imagefile'); % Use "Edit Image" on toolstrip to change.
  v_float_D : Outport
  v_float_Q : Outport  Port=2
  wires:
  line charging dynamics/1(v_float_D) -> v_float_D/1
  line charging dynamics/2(v_float_Q) -> v_float_Q/1
  In1/1 -> i_float_D/1
  i_float_Q/1 -> line charging dynamics/2(i_float_Q)
  In2/1 -> i_float_Q/1
  i_float_D/1 -> line charging dynamics/1(i_float_D)

== system subsystem_118_bus/Subsystem2/area2/non_ibr/infinite bus ==
  v_inf_D : Constant  Value=Subsystem.infbus.v_D
  v_inf_Q : Constant  Value=Subsystem.infbus.v_Q
  Out1 : Outport
  Out2 : Outport  Port=2
  wires:
  v_inf_D/1 -> Out1/1
  v_inf_Q/1 -> Out2/1

== system subsystem_118_bus/Subsystem2/area2/non_ibr/load buses ==
  In1 : Inport
  In2 : Inport  Port=2
  Constant : Constant  Value=Subsystem.load1.v_D
  Constant1 : Constant  Value=Subsystem.load1.v_Q
  Constant2 : Constant  Value=Subsystem.load1.ptype
  Constant3 : Constant  Value=Subsystem.load1.qtype
  Divide : Product  Inputs=*/
  Product : Product
  Product1 : Product
  Sqrt : Sqrt
  Sqrt1 : Sqrt
  Square1 : Math  Operator=pow
  Square{2..5} (4 alike) : Math  Operator=square
  Square6 : Math  Operator=pow
  Subsystem : Subsystem
  Sum : Sum  Inputs=|-+
  Sum1 : Sum  Inputs=|-+
  Sum2 : Sum
  Sum4 : Sum
  i_load_D : Selector  InputPortWidth=size(Subsystem.sys_data,1)  IndexOptions=Index vector (dialog)  Indices=Subsystem.busnum.load  OutputSizes=1
  i_load_Q : Selector  InputPortWidth=size(Subsystem.sys_data,1)  IndexOptions=Index vector (dialog)  Indices=Subsystem.busnum.load  OutputSizes=1
  line charging dynamics : Subsystem
      mask Display: image('$imagefile'); % Use "Edit Image" on toolstrip to change.
  load bus p : Constant  Value=Subsystem.load1.p
  load bus q : Constant  Value=Subsystem.load1.q
  Out1 : Outport
  Out2 : Outport  Port=2
  wires:
  Constant3/1 -> Square1/2
  [v_load_Q] -> Square5/1
  Square2/1 -> Sum4/1
  Sum4/1 -> Sqrt/1
  Sqrt1/1 -> Divide/1
  Square3/1 -> Sum4/2
  Sqrt/1 -> Divide/2
  Constant/1 -> Square2/1
  Divide/1 -> Square1/1, Square6/1
  Constant2/1 -> Square6/2
  Square5/1 -> Sum2/2
  [v_load_D] -> Square4/1
  Constant1/1 -> Square3/1
  Square4/1 -> Sum2/1
  Sum2/1 -> Sqrt1/1
  Square1/1 -> Product1/1
  line charging dynamics/2(v_load_Q) -> [v_load_Q], Out2/1
  line charging dynamics/1(v_load_D) -> [v_load_D], Out1/1
  load bus q/1 -> Product1/2
  Product1/1 -> Subsystem/2(q)
  Product/1 -> Subsystem/1(p)
  Square6/1 -> Product/2
  load bus p/1 -> Product/1
  Sum/1 -> line charging dynamics/1(i_load_c_D)
  Subsystem/1(i_inj_load_d) -> Sum/2
  Subsystem/2(i_inj_load_q) -> Sum1/2
  [v_load_Q] -> Subsystem/4(vQ)
  [v_load_D] -> Subsystem/3(vD)
  i_load_D/1 -> Sum/1
  i_load_Q/1 -> Sum1/1
  Sum1/1 -> line charging dynamics/2(i_load_c_Q)
  In2/1 -> i_load_Q/1
  In1/1 -> i_load_D/1

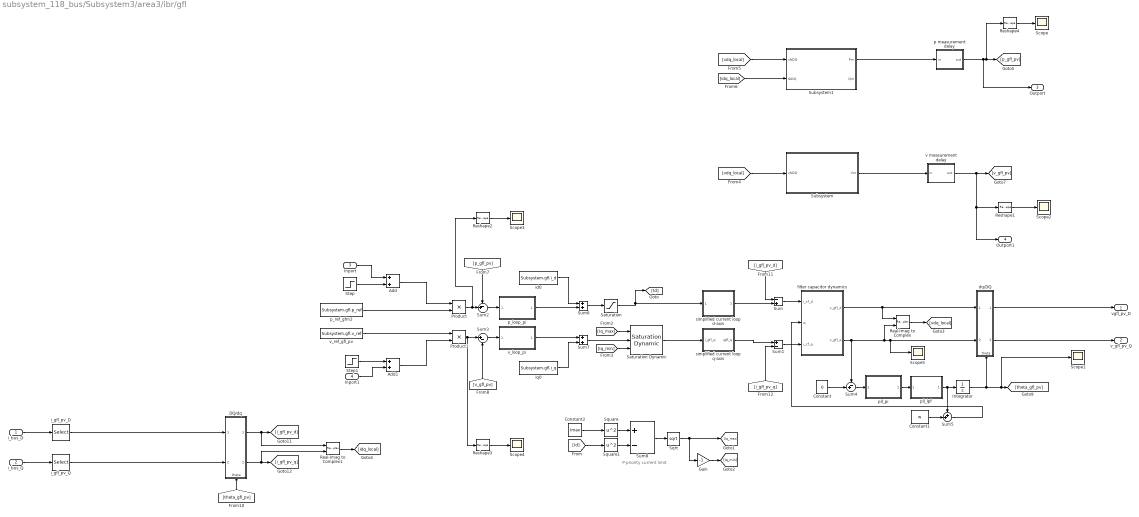
== system subsystem_118_bus/Subsystem3/area3/ibr/gfl ==
  note: P-priority current limit
  i_bus_D : Inport
  i_bus_Q : Inport  Port=2
  Inport : Inport  Port=3
  Inport1 : Inport  Port=4
  Add : Sum
  Add1 : Sum
  Constant : Constant  Value=0
  Constant1 : Constant  Value=w
  Constant2 : Constant  Value=Imax
  DQ/dq : Subsystem
      settings: PortSchema="{\"entries\":[{\"content\":{\"sides\":[{\"content\":{\"connectorIds\":[\"In1\",\"In2\"]},\"type\":\"ConnectorPlacement.EquallySpacedRectSide\",\"uuid\":\"6aba5a73-e9d3-440a-9da8-5b4060b79a22\"},{\"content\":{\"connectorIds\":[\"Out1\",\"Out2\"],\"side\":\"RIGHT\"},\"type\":\"ConnectorPlacement.EquallySpacedRectSide\",\"uuid\":\"fb100e33-0f2b-446b-b234-6a01cff1cf94\"},{\"content\":{\"connectorIds\":[],\"side\":\"TOP\"},\"type\":\"ConnectorPlacement.EquallySpacedRectSide\",\"uuid\":\"cb346bab-8363-4920-b8bd-1af08716b150\"},{\"content\":{\"connectorIds\":[\"In3\"],\"side\":\"BOTTOM\"},\"type\":\"ConnectorPlacement.EquallySpacedRectSide\",\"uuid\":\"daf67601-a33f-44c6-bbbf-d32eadf086e5\"},{\"content\":{\"connectorIds\":[],\"side\":\"HIDDEN\"},\"type\":\"ConnectorPlacement.EquallySpacedRectSide\",\"uuid\":\"157b31a2-d1ec-4854-8b21-1495795af5ef\"}]},\"type\":\"ConnectorPlacement.EquallySpacedConnector\",\"uuid\":\"bdcd0df2-60ef-4202-9e13-560935cf5e64\"}],\"packageUris\":[\"http://schema.mathworks.com/mf0/Connector/R2020b\"],\"version\":\"1.0\"}"
      mask Display: image('$imagefile'); % Use "Edit Image" on toolstrip to change.
  Gain : Gain  Gain=-1
  Integrator : Integrator  InitialCondition=Subsystem.gfl.theta  ContinuousStateAttributes='gfl_osc'
  Product : Product
  Product1 : Product
  Real-Imag to Complex : RealImagToComplex
  Real-Imag to Complex1 : RealImagToComplex
  Reshape{1..4} (4 alike) : Reshape
  Saturation : Saturate  UpperLimit=Imax  LowerLimit=-Imax
  Saturation Dynamic : simulink/Discontinuities/Saturation Dynamic  OutMin=[]  OutMax=[]  OutDataTypeStr=Inherit: Same as second input  OutDataType=fixdt(1, 16)  OutScaling=2^-10  DoSatur=off
  Scope{,1..5} (6 alike) : Scope
      Scope settings: ActiveDisplayYMinimum=-1  ActiveDisplayYMaximum=1  DataLoggingVariableName=pm_gfl  DataLoggingSaveFormat=Structure
      Scope1 settings: ActiveDisplayYMinimum=-0.38233203386380687  ActiveDisplayYMaximum=-0.24913479990794113  DataLoggingVariableName=thetagflwnd  DataLoggingSaveFormat=Structure
      Scope2 settings: ActiveDisplayYMinimum=-1  ActiveDisplayYMaximum=1  DataLoggingVariableName=vm_gfl  DataLoggingSaveFormat=Structure
      Scope3 settings: ActiveDisplayYMinimum=-0.062499999999999986  ActiveDisplayYMaximum=0.5625  DataLoggingVariableName=pr_gfl  DataLoggingSaveFormat=Structure
      Scope4 settings: ActiveDisplayYMinimum=1.02188  ActiveDisplayYMaximum=1.05312  DataLoggingVariableName=vr_gfl  DataLoggingSaveFormat=Structure
      Scope5 settings: DataLoggingVariableName=ScopeData3
  Sqrt : Sqrt
  Square : Math  Operator=square
  Square1 : Math  Operator=square
  Step : Step  Time=Tstep_gfl  Before=Subsystem.P_before_gfl  After=Subsystem.P_after_gfl  SampleTime=0
  Step1 : Step  Time=Tstep_gfl  Before=Subsystem.V_before_gfl  After=Subsystem.V_after_gfl  SampleTime=0
  Subsystem : Subsystem
      mask Display: image('$imagefile'); % Use "Edit Image" on toolstrip to change.
  Subsystem1 : Subsystem
      mask Display: image('$imagefile'); % Use "Edit Image" on toolstrip to change.
  Sum : Sum  Inputs=-+
  Sum1 : Sum  Inputs=+-
  Sum2 : Sum  Inputs=-+|
  Sum3 : Sum  Inputs=|+-
  Sum4 : Sum  Inputs=-+|
  Sum5 : Sum  Inputs=++|
  Sum6 : Sum
  Sum7 : Sum
  Sum8 : Sum  Inputs=+-
  dq/DQ : Subsystem
      settings: PortSchema="{\"entries\":[{\"content\":{\"sides\":[{\"content\":{\"connectorIds\":[\"In1\",\"In2\"]},\"type\":\"ConnectorPlacement.EquallySpacedRectSide\",\"uuid\":\"6aba5a73-e9d3-440a-9da8-5b4060b79a22\"},{\"content\":{\"connectorIds\":[\"Out1\",\"Out2\"],\"side\":\"RIGHT\"},\"type\":\"ConnectorPlacement.EquallySpacedRectSide\",\"uuid\":\"fb100e33-0f2b-446b-b234-6a01cff1cf94\"},{\"content\":{\"connectorIds\":[],\"side\":\"TOP\"},\"type\":\"ConnectorPlacement.EquallySpacedRectSide\",\"uuid\":\"cb346bab-8363-4920-b8bd-1af08716b150\"},{\"content\":{\"connectorIds\":[\"In3\"],\"side\":\"BOTTOM\"},\"type\":\"ConnectorPlacement.EquallySpacedRectSide\",\"uuid\":\"daf67601-a33f-44c6-bbbf-d32eadf086e5\"},{\"content\":{\"connectorIds\":[],\"side\":\"HIDDEN\"},\"type\":\"ConnectorPlacement.EquallySpacedRectSide\",\"uuid\":\"157b31a2-d1ec-4854-8b21-1495795af5ef\"}]},\"type\":\"ConnectorPlacement.EquallySpacedConnector\",\"uuid\":\"bdcd0df2-60ef-4202-9e13-560935cf5e64\"}],\"packageUris\":[\"http://schema.mathworks.com/mf0/Connector/R2020b\"],\"version\":\"1.0\"}"
      mask Display: image('$imagefile'); % Use "Edit Image" on toolstrip to change.
  filter capacitor dynamics : Subsystem
      mask Display: image('$imagefile'); % Use "Edit Image" on toolstrip to change.
  i_gfl_pv_D : Selector  InputPortWidth=size(Subsystem.sys_data,1)  IndexOptions=Index vector (dialog)  Indices=Subsystem.busnum.gfl  OutputSizes=1
  i_gfl_pv_Q : Selector  InputPortWidth=size(Subsystem.sys_data,1)  IndexOptions=Index vector (dialog)  Indices=Subsystem.busnum.gfl  OutputSizes=1
  id0 : Constant  Value=Subsystem.gfl.i_d
  iq0 : Constant  Value=Subsystem.gfl.i_q
  p measurement delay : Subsystem
      mask Display: image('$imagefile'); % Use "Edit Image" on toolstrip to change.
  p_loop_pi : Subsystem
      mask Display: image('$imagefile'); % Use "Edit Image" on toolstrip to change.
  p_ref_gfm2 : Constant  Value=Subsystem.gfl.p_ref
  pll_lpf : Subsystem
      mask Display: image('$imagefile'); % Use "Edit Image" on toolstrip to change.
  pll_pi : Subsystem
      mask Display: image('$imagefile'); % Use "Edit Image" on toolstrip to change.
  simplified current loop d-axis : Subsystem
      mask Display: image('$imagefile'); % Use "Edit Image" on toolstrip to change.
  simplified current loop q-axis : Subsystem
      mask Display: image('$imagefile'); % Use "Edit Image" on toolstrip to change.
  v measurement delay : Subsystem
      mask Display: image('$imagefile'); % Use "Edit Image" on toolstrip to change.
  v_loop_pi : Subsystem
      mask Display: image('$imagefile'); % Use "Edit Image" on toolstrip to change.
  v_ref_gfl_pv : Constant  Value=Subsystem.gfl.v_ref
  vgfl_pv_D : Outport
  v_gfl_pv_Q : Outport  Port=2
  Outport : Outport  Port=3
  Outport1 : Outport  Port=4
  wires:
  pll_lpf/1(LPF_output) -> Sum5/1, Integrator/1
  Constant/1 -> Sum4/2
  filter capacitor dynamics/1(v_gfl_d) -> dq/DQ/1(d-quantity), Real-Imag to Complex/1
  v measurement delay/1(out) -> Reshape1/1, Outport1/1, [v_gfl_pv]
  filter capacitor dynamics/2(v_gfl_q) -> Real-Imag to Complex/2, Scope5/1, dq/DQ/2(q-quantity), Sum4/1
  [p_gfl_pv] -> Sum2/1
  Sum1/1 -> filter capacitor dynamics/3(i_cf_q)
  Sum4/1 -> pll_pi/1("  ")
  Sum5/1 -> filter capacitor dynamics/2(w)
  dq/DQ/1(D-quantity) -> vgfl_pv_D/1
  Sum2/1 -> p_loop_pi/1("  ")
  p measurement delay/1(out) -> Outport/1, Reshape4/1, [p_gfl_pv]
  Constant1/1 -> Sum5/2
  Sum3/1 -> v_loop_pi/1("  ")
  [i_gfl_pv_d] -> Sum/1
  Sum/1 -> filter capacitor dynamics/1(i_cf_d)
  [i_gfl_pv_q] -> Sum1/2
  [theta_gfl_pv] -> DQ/dq/3(theta)
  pll_pi/1(" ") -> pll_lpf/1(LPF_input)
  [v_gfl_pv] -> Sum3/2
  i_bus_Q/1 -> i_gfl_pv_Q/1
  i_bus_D/1 -> i_gfl_pv_D/1
  p_loop_pi/1(" ") -> Sum6/2
  v_loop_pi/1(" ") -> Sum7/1
  iq0/1 -> Sum7/2
  id0/1 -> Sum6/1
  Sum6/1 -> Saturation/1
  Integrator/1 -> Scope1/1, [theta_gfl_pv], dq/DQ/3(theta)
  Reshape4/1 -> Scope/1
  Reshape1/1 -> Scope2/1
  [Id] -> Square1/1
  Gain/1 -> [Iq_min]
  Constant2/1 -> Square/1
  Square/1 -> Sum8/1
  Sqrt/1 -> [Iq_max], Gain/1
  Square1/1 -> Sum8/2
  Sum8/1 -> Sqrt/1
  Saturation/1 -> simplified current loop d-axis/1(" "), [Id]
  Sum7/1 -> Saturation Dynamic/2
  [Iq_max] -> Saturation Dynamic/1
  [Iq_min] -> Saturation Dynamic/3
  simplified current loop d-axis/1("  ") -> Sum/2
  Saturation Dynamic/1 -> simplified current loop q-axis/1(i_gfl_q)
  simplified current loop q-axis/1(igfl_q) -> Sum1/1
  [vdq_local] -> Subsystem/1(vbDQ)
  [vdq_local] -> Subsystem1/1(vbDQ)
  [idq_local] -> Subsystem1/2(IbDQ)
  Real-Imag to Complex/1 -> [vdq_local]
  DQ/dq/1(d_quantity) -> Real-Imag to Complex1/1, [i_gfl_pv_d]
  DQ/dq/2(q_quantity) -> Real-Imag to Complex1/2, [i_gfl_pv_q]
  Real-Imag to Complex1/1 -> [idq_local]
  dq/DQ/2(Q-quantity) -> v_gfl_pv_Q/1
  Subsystem/1(Vm) -> v measurement delay/1(in)
  Subsystem1/1(Pm) -> p measurement delay/1(in)
  p_ref_gfm2/1 -> Product/2
  v_ref_gfl_pv/1 -> Product1/1
  Reshape2/1 -> Scope3/1
  Product/1 -> Reshape2/1, Sum2/2
  Reshape3/1 -> Scope4/1
  Product1/1 -> Sum3/1, Reshape3/1
  Step/1 -> Add/2
  Add/1 -> Product/1
  Step1/1 -> Add1/1
  Add1/1 -> Product1/2
  Inport/1 -> Add/1
  Inport1/1 -> Add1/2
  i_gfl_pv_D/1 -> DQ/dq/1(D_quantity)
  i_gfl_pv_Q/1 -> DQ/dq/2(Q_quantity)
